simulink model "final_gyro_compass"  (R2022b)
settings: Solver=FixedStepAuto  StartTime=0.0  StopTime=10.0  FixedStep=0.01  MaxStep=0.01  RelTol=1e-3
libraries: dspxfrm3 x1
settings Model: Creator=zd012  LastModifiedBy=zd012
settings DebuggingCC: UnconnectedInputMsg=warning  UnconnectedOutputMsg=warning  UnconnectedLineMsg=warning
settings ModelReferenceCC: EnableRefExpFcnMdlSchedulingChecks=on
settings RTWCC: DLArmComputeVersion=19.05

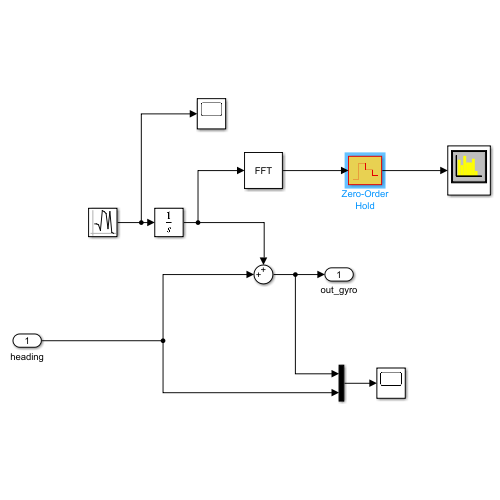
[thumbnail: Simulink's stored preview of the top-level diagram]
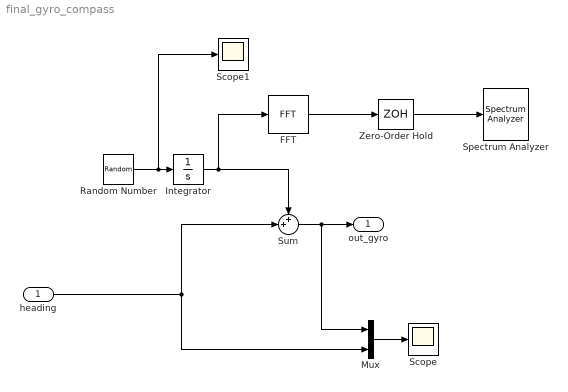
== system final_gyro_compass ==
  heading : Inport
  FFT : dspxfrm3/FFT  FFTImplementation=Auto  CompMethod=Table lookup  TableOpt=NEW  TableOptActive=Speed  BitRevOrder=off  Normalize=off  InheritFFTLength=on  FFTLength=64  WrapInput=on  roundingMode=Floor  overflowMode=off  firstCoeffDataTypeStr=Inherit: Same word length as input  firstCoeffLastDataTypeStr=Inherit: Same word length as input  outputMin=[]  outputMax=[]
  Integrator : Integrator
  Mux : Mux  Inputs=2
  Random Number : RandomNumber  Mean=0.02  Variance=0.01  SampleTime=0.1
  Scope : Scope
  Scope1 : Scope
  Spectrum Analyzer : SpectrumAnalyzer
  Sum : Sum  Inputs=++|
  Zero-Order Hold : ZeroOrderHold  SampleTime=-1
  out_gyro : Outport
  wires:
  Random Number/1 -> Scope1/1, Integrator/1
  Integrator/1 -> FFT/1, Sum/1
  heading/1 -> Mux/2, Sum/2
  Sum/1 -> Mux/1, out_gyro/1
  Zero-Order Hold/1 -> Spectrum Analyzer/1
  Mux/1 -> Scope/1
  FFT/1 -> Zero-Order Hold/1
